simulink model "ESP32_CONTROL_SYSTEM"  (R2024a)
settings: Solver=FixedStepAuto  StartTime=0.0  StopTime=inf  FixedStep=0.05  RelTol=1e-3
values from neighbouring files (symbols this model uses):
  Beta1 = 3*Omega_o    (= 150)    [ESP32_ANALOG_READ_VAR.m]
  Beta2 = 3*(Omega_o^2)    (= 7500)    [ESP32_ANALOG_READ_VAR.m]
  Beta3 = (Omega_o^3)    (= 125000)    [ESP32_ANALOG_READ_VAR.m]
  Desire_Max = 255    [ESP32_ANALOG_READ_VAR.m]
  Desire_Min = 0    [ESP32_ANALOG_READ_VAR.m]
  Direction_Pin = 0    [ESP32_ANALOG_READ_VAR.m]
  EN_Pin = 1    [ESP32_ANALOG_READ_VAR.m]
  J_aet = 0.0035    [ESP32_ANALOG_READ_VAR.m]
  Kd = 1    [ESP32_ANALOG_READ_VAR.m]
  Ki = 2    [ESP32_ANALOG_READ_VAR.m]
  Kp = 3    [ESP32_ANALOG_READ_VAR.m]
  omga_c = 2    [ESP32_ANALOG_READ_VAR.m]
  roa = 0.24    [ESP32_ANALOG_READ_VAR.m]
libraries: arduinolib x6, simulink_extras x5, simulink x1
(part 3 of 3)

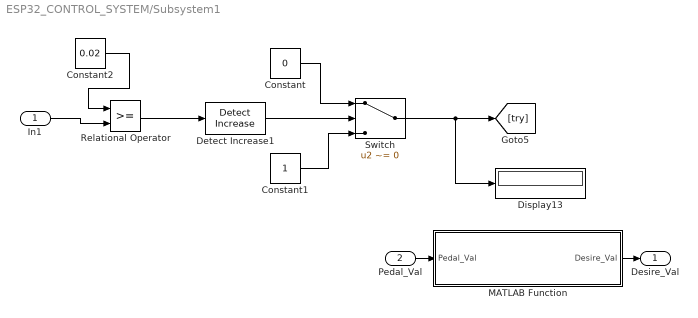
== system ESP32_CONTROL_SYSTEM/Subsystem1 ==
  In1 : Inport
  Pedal_Val : Inport  Port=2
  Constant : Constant  Value=0
  Constant1 : Constant
  Constant2 : Constant  Value=0.02
  Detect Increase1 : simulink/Logic and Bit Operations/Detect Increase  vinit=0.0  OutDataTypeStr=boolean
  Display13 : Display
      settings: Decimation=2
  MATLAB Function : MATLAB Function  TreatAsAtomicUnit=on
  Relational Operator : RelationalOperator  OutDataTypeStr=boolean  RndMeth=Simplest  InputSameDT=off
  Switch : Switch  Criteria=u2 ~= 0  Threshold=1  SaturateOnIntegerOverflow=off  InputSameDT=off
  Desire_Val : Outport
  wires:
  MATLAB Function/1(Desire_Val) -> Desire_Val/1
  In1/1 -> Relational Operator/2
  Switch/1 -> Display13/1, [try]
  Detect Increase1/1 -> Switch/2
  Constant/1 -> Switch/1
  Constant2/1 -> Relational Operator/1
  Constant1/1 -> Switch/3
  Relational Operator/1 -> Detect Increase1/1
  Pedal_Val/1 -> MATLAB Function/1(Pedal_Val)

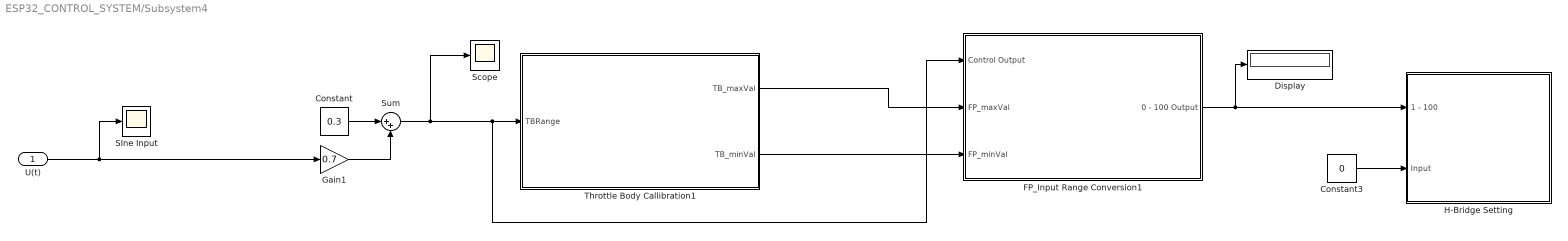
== system ESP32_CONTROL_SYSTEM/Subsystem4 ==
  U(t) : Inport
  Constant : Constant  Value=0.3
  Constant3 : Constant  Value=0
  Display : Display
  FP_Input Range Conversion1 : Subsystem
  Gain1 : Gain  Gain=0.7
  H-Bridge Setting : Subsystem
      mask Display: image('H-Bridge.JPG');
  SIne Input : Scope
  Scope : Scope
  Sum : Sum  Inputs=|++
  Throttle Body Callibration1 : MATLAB Function  TreatAsAtomicUnit=on
  wires:
  Constant/1 -> Sum/1
  FP_Input Range Conversion1/1(0 - 100 Output) -> Display/1, H-Bridge Setting/1(1 - 100)
  Constant3/1 -> H-Bridge Setting/2(Input)
  Sum/1 -> Scope/1, FP_Input Range Conversion1/1(Control Output), Throttle Body Callibration1/1(TBRange)
  Throttle Body Callibration1/2(TB_minVal) -> FP_Input Range Conversion1/3(FP_minVal)
  Gain1/1 -> Sum/2
  U(t)/1 -> SIne Input/1, Gain1/1
  Throttle Body Callibration1/1(TB_maxVal) -> FP_Input Range Conversion1/2(FP_maxVal)

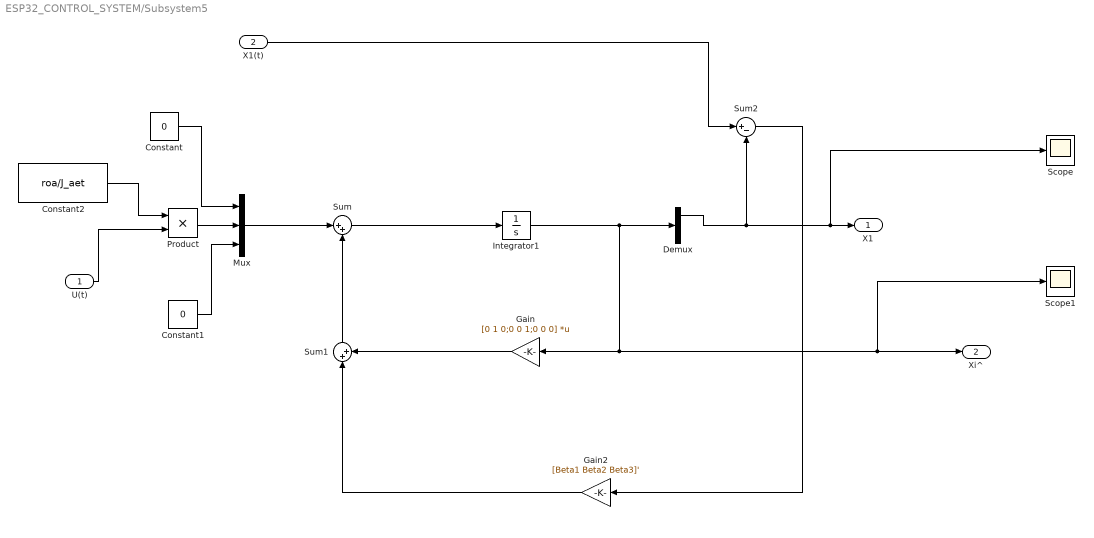
== system ESP32_CONTROL_SYSTEM/Subsystem5 ==
  U(t) : Inport
  X1(t) : Inport  Port=2
  Constant : Constant  Value=0
  Constant1 : Constant  Value=0
  Constant2 : Constant  Value=roa/J_aet
  Demux : Demux  Outputs=3
  Gain : Gain  Gain=[0 1 0;0 0 1;0 0 0]  Multiplication=Matrix(K*u)
  Gain2 : Gain  Gain=[Beta1 Beta2 Beta3]'
  Integrator1 : Integrator  InitialCondition=[12*pi/180 0 0]'
  Mux : Mux  Inputs=3
  Product : Product  RndMeth=Zero
  Scope : Scope
  Scope1 : Scope
  Sum : Sum  Inputs=|++
  Sum1 : Sum  Inputs=|++
  Sum2 : Sum  Inputs=|+-
  X1 : Outport
  Xi^ : Outport  Port=2
  wires:
  Integrator1/1 -> Gain/1, Xi^/1, Scope1/1, Demux/1
  Sum/1 -> Integrator1/1
  Product/1 -> Mux/2
  Constant2/1 -> Product/1
  U(t)/1 -> Product/2
  Gain/1 -> Sum1/2
  Constant/1 -> Mux/1
  Constant1/1 -> Mux/3
  Mux/1 -> Sum/1
  Sum1/1 -> Sum/2
  Demux/1 -> Sum2/2, X1/1, Scope/1
  X1(t)/1 -> Sum2/1
  Sum2/1 -> Gain2/1
  Gain2/1 -> Sum1/1

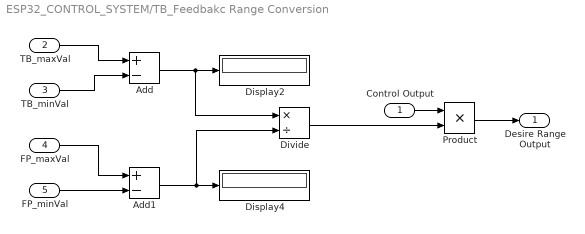
== system ESP32_CONTROL_SYSTEM/TB_Feedbakc Range Conversion ==
  Control Output : Inport
  TB_maxVal : Inport  Port=2
  TB_minVal : Inport  Port=3
  FP_maxVal : Inport  Port=4
  FP_minVal : Inport  Port=5
  Add : Sum  Inputs=+-
  Add1 : Sum  Inputs=+-
  Display2 : Display
  Display4 : Display
  Divide : Product  Inputs=*/
  Product : Product
  " Desire Range Output" : Outport
  wires:
  Product/1 -> " Desire Range Output"/1
  Control Output/1 -> Product/1
  Divide/1 -> Product/2
  Add1/1 -> Display4/1, Divide/2
  Add/1 -> Display2/1, Divide/1
  TB_maxVal/1 -> Add/1
  TB_minVal/1 -> Add/2
  FP_maxVal/1 -> Add1/1
  FP_minVal/1 -> Add1/2

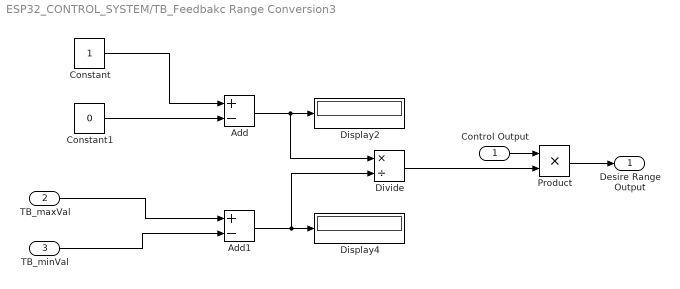
== system ESP32_CONTROL_SYSTEM/TB_Feedbakc Range Conversion3 ==
  Control Output : Inport
  TB_maxVal : Inport  Port=2
  TB_minVal : Inport  Port=3
  Add : Sum  Inputs=+-
  Add1 : Sum  Inputs=+-
  Constant : Constant
  Constant1 : Constant  Value=0
  Display2 : Display
  Display4 : Display
  Divide : Product  Inputs=*/
  Product : Product
  " Desire Range Output" : Outport
  wires:
  Add/1 -> Divide/1, Display2/1
  Add1/1 -> Divide/2, Display4/1
  Divide/1 -> Product/2
  Control Output/1 -> Product/1
  Product/1 -> " Desire Range Output"/1
  Constant/1 -> Add/1
  Constant1/1 -> Add/2
  TB_maxVal/1 -> Add1/1
  TB_minVal/1 -> Add1/2

== system ESP32_CONTROL_SYSTEM/Throttle Body  ==
  ESP23_ANALOG_READ_DDAppGeneratedBlock : MATLABSystem  System=ESP32_ANALOG_READ  PIN=int8( 35 )  SampleTime=-1
      mask Type: ESP32_ANALOG_READ
      mask Display:
      | color('white');plot([100,100,100,100]*1,[100,100,100,100]*1);plot([100,100,100,100]*0,[100,100,100,100]*0);color('blue');text(38, 92, 'IO Device Builder','horizontalAlignment', 'right');
      | color('black');text(52,50,' ESP32_ANALOG_READ','horizontalAlignment','center');
      | port_label('output',1,'V');
  Throttle Body Feedback : Outport
  wires:
  ESP23_ANALOG_READ_DDAppGeneratedBlock/1 -> Throttle Body Feedback/1

== system ESP32_CONTROL_SYSTEM/Throttle Body Feedback1 ==
  ESP23_ANALOG_READ_DDAppGeneratedBlock : MATLABSystem  System=ESP32_ANALOG_READ  PIN=int8( 35 )  SampleTime=-1
      mask Type: ESP32_ANALOG_READ
      mask Display:
      | color('white');plot([100,100,100,100]*1,[100,100,100,100]*1);plot([100,100,100,100]*0,[100,100,100,100]*0);color('blue');text(38, 92, 'IO Device Builder','horizontalAlignment', 'right');
      | color('black');text(52,50,' ESP32_ANALOG_READ','horizontalAlignment','center');
      | port_label('output',1,'V');
  Out1 : Outport
  wires:
  ESP23_ANALOG_READ_DDAppGeneratedBlock/1 -> Out1/1

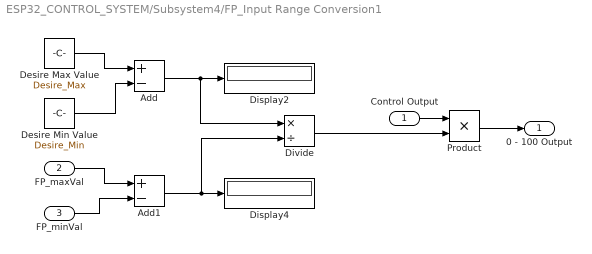
== system ESP32_CONTROL_SYSTEM/Subsystem4/FP_Input Range Conversion1 ==
  Control Output : Inport
  FP_maxVal : Inport  Port=2
  FP_minVal : Inport  Port=3
  Add : Sum  Inputs=+-
  Add1 : Sum  Inputs=+-
  Desire Max Value : Constant  Value=Desire_Max
  Desire Min Value : Constant  Value=Desire_Min
  Display2 : Display
  Display4 : Display
  Divide : Product  Inputs=*/
  Product : Product
  0 - 100 Output : Outport
  wires:
  FP_maxVal/1 -> Add1/1
  Product/1 -> 0 - 100 Output/1
  Control Output/1 -> Product/1
  Desire Min Value/1 -> Add/2
  Divide/1 -> Product/2
  Desire Max Value/1 -> Add/1
  Add1/1 -> Display4/1, Divide/2
  FP_minVal/1 -> Add1/2
  Add/1 -> Display2/1, Divide/1

== system ESP32_CONTROL_SYSTEM/Subsystem4/H-Bridge Setting ==
  1 - 100 : Inport
  Input : Inport  Port=2
  Digital Output : arduinolib/Digital Output  pinNumber=4  Direction=output  blockPlatform=arduino
  Digital Output1 : arduinolib/Digital Output  pinNumber=0  Direction=output  blockPlatform=arduino
  Display3 : Display
  Display4 : Display
  Enable Pin : Constant  Value=EN_Pin
  PWM : arduinolib/PWM  pinNumber=2  frequencyType=Specify  desiredFrequency=19000  achievableFrequency=19000
  wires:
  Enable Pin/1 -> Display4/1, Digital Output/1
  1 - 100/1 -> PWM/1
  Input/1 -> Display3/1, Digital Output1/1

== matlab function ESP32_CONTROL_SYSTEM/Pedal Calibration ==
  settings: updateMethod=DISCRETE
  data: PedalRange input; FP_maxVal output; FP_minVal output
function [FP_maxVal, FP_minVal] = FootPadel_Range(PedalRange)
    persistent maxSet minSet;
    if isempty(maxSet)
        maxSet = -1;
    end
    if isempty(minSet)
        minSet = 5; 
    end
    if PedalRange > maxSet
        maxSet = PedalRange;
    end
    if PedalRange < minSet
        minSet = PedalRange;
    end
    FP_maxVal = maxSet;
    FP_minVal = minSet;
end

== matlab function ESP32_CONTROL_SYSTEM/Subsystem1/MATLAB Function ==
  data: Pedal_Val input; Desire_Val output
function Desire_Val = fcn(Pedal_Val)

persistent Previous_Val Set_Val
if isempty(Set_Val)
    Set_Val = 0;
end
if isempty(Previous_Val)
    Previous_Val = 0;
else
    Set_Val = abs(Previous_Val - Pedal_Val);
    Previous_Val = Pedal_Val;
end
Desire_Val = abs(Set_Val);
end

== matlab function ESP32_CONTROL_SYSTEM/Throttle Body Callibration1 ==
  settings: updateMethod=DISCRETE
  data: TBRange input; TB_maxVal output; TB_minVal output
function [TB_maxVal, TB_minVal] = ThrottleBody_Range(TBRange)
    persistent TB_maxSet TB_minSet;
    if isempty(TB_maxSet)
        TB_maxSet = 0;
    end
    if isempty(TB_minSet)
        TB_minSet = 5; 
    end
    if TBRange > TB_maxSet
        TB_maxSet = TBRange;
    end
    if TBRange < TB_minSet
        TB_minSet = TBRange;
    end
    TB_maxVal = TB_maxSet;
    TB_minVal = TB_minSet;
end

== matlab function ESP32_CONTROL_SYSTEM/Subsystem4/Throttle Body Callibration1 ==
  settings: updateMethod=DISCRETE
  data: TBRange input; TB_maxVal output; TB_minVal output
function [TB_maxVal, TB_minVal] = ThrottleBody_Range(TBRange)
    persistent TB_maxSet TB_minSet;
    if isempty(TB_maxSet)
        TB_maxSet = 0;
    end
    if isempty(TB_minSet)
        TB_minSet = 5; 
    end
    if TBRange > TB_maxSet
        TB_maxSet = TBRange;
    end
    if TBRange < TB_minSet
        TB_minSet = TBRange;
    end
    TB_maxVal = TB_maxSet;
    TB_minVal = TB_minSet;
end

== matlab function ESP32_CONTROL_SYSTEM/Throttle Body Callibration ==
  settings: updateMethod=DISCRETE
  data: TBRange input; TB_maxVal output; TB_minVal output
function [TB_maxVal, TB_minVal] = ThrottleBody_Range(TBRange)
    persistent TB_maxSet TB_minSet;
    if isempty(TB_maxSet)
        TB_maxSet = 0;
    end
    if isempty(TB_minSet)
        TB_minSet = 5; 
    end
    if TBRange > TB_maxSet
        TB_maxSet = TBRange;
    end
    if TBRange < TB_minSet
        TB_minSet = TBRange;
    end
    TB_maxVal = TB_maxSet;
    TB_minVal = TB_minSet;
end
